simulink model "MOBATSim"  (R2020b)
settings: Solver=FixedStepAuto  StartTime=0.0  StopTime=Sim_t  FixedStep=0.01  MinStep=0.01  RelTol=1e-2
undefined symbols (not defined in the file): meters, noisePower, Sim_Ts, stuckDuration, Vehicle_id, Vehicles
libraries: simulink x32, robotalgslib x11, drivingvehiclecontroller x11, mpcadaslib x1, pid_lib x1
(part 2 of 5)

== system MOBATSim/Vehicle Model 8 ==
  note: Perception
  note: Decision-Making
  note: Control
  Behavioural Planner : MATLABSystem  System=VehicleDrivingMode  Vehicle_id=Vehicle_id  SimulateUsing=Interpreted execution
      mask Type: VehicleDrivingMode
      mask Display:
      | image('MOBATSIM-Icon-Set_7- Behavioural Planner.png');
      | port_label('input',1,'vehicleDetected');
      | port_label('output',1,'SpeedReference');
      | port_label('output',2,'DistanceReference');
      | port_label('output',3,'LeadSpeed');
      | port_label('output',4,'DrivingMode');
      | port_label('output',5,'Dist2Stop');
      | port_label('output',6,'laneChange');
  Longitudinal and Lateral Controllers : Subsystem
  Safety Filter : Subsystem
  Transform to MOBATSim Coordinates : Subsystem
  Vehicle Model - Kinematic 3DOF Single Track : Subsystem  mask{Vehicle_id=Vehicle_id}
      mask prompts: Vehicle_id "Vehicle ID"
      mask Display: image('MOBATSIM-Icon-Set_13- VehicleModel.png'); % Use "Edit Image" on toolstrip to change.
  Vehicle Path Planner : MATLABSystem  System=VehiclePathPlanner_Astar  Vehicle_id=Vehicle_id  SimulateUsing=Interpreted execution
      mask Type: VehiclePathPlanner_Astar
      mask Display:
      | image('MOBATSIM-Icon-Set_8- Navigation.png');
      | port_label('input',1,'CommunicationIDs');
      | port_label('output',1,'waypointReached');
  Vehicle Sensors : MATLABSystem  System=VehicleSensors  Vehicle_id=Vehicle_id  Tsample=Sim_Ts  OffsetTime=0  SimulateUsing=Interpreted execution
      mask Type: VehicleSensors
      mask Display:
      | image('MOBATSIM-Icon-Set_4- Sensor.png');
      | port_label('output',1,'V2VcommIDs');
      | port_label('output',2,'vehicleDetected');
  Vehicle V2I Output : MATLABSystem  System=VehicleV2I_Out  Vehicle_id=Vehicle_id  SimulateUsing=Interpreted execution
      mask Type: VehicleV2I_Out
      mask Display:
      | image('MOBATSIM-Icon-Set_6- V2l.png');
      | port_label('input',1,'waypointReached');
      | port_label('output',1,'V2Idata');
  Position : Outport  VectorParamsAs1DForOutWhenUnconnected=off
  Orientation : Outport  Port=2  VectorParamsAs1DForOutWhenUnconnected=off
  Speed : Outport  Port=3  VectorParamsAs1DForOutWhenUnconnected=off
  V_Network_Out : Outport  Port=4  VectorParamsAs1DForOutWhenUnconnected=off
  wires:
  Vehicle Path Planner/1 -> Vehicle V2I Output/1
  Vehicle Sensors/1 -> Vehicle Path Planner/1
  Vehicle V2I Output/1 -> V_Network_Out/1
  Vehicle Sensors/2 -> Behavioural Planner/1
  Behavioural Planner/1 -> Longitudinal and Lateral Controllers/1(Speed Reference)
  Behavioural Planner/2 -> Longitudinal and Lateral Controllers/2(Inter Vehicular Distance)
  Behavioural Planner/3 -> Longitudinal and Lateral Controllers/3(Lead Speed)
  Behavioural Planner/4 -> Longitudinal and Lateral Controllers/4(drivingMode)
  Behavioural Planner/5 -> Longitudinal and Lateral Controllers/5(Dist2Stop)
  Transform to MOBATSim Coordinates/1(Position) -> Position/1
  Transform to MOBATSim Coordinates/2(Orientation) -> Orientation/1
  Vehicle Model - Kinematic 3DOF Single Track/2(xdot) -> Longitudinal and Lateral Controllers/7(Actual Speed), Speed/1
  Vehicle Model - Kinematic 3DOF Single Track/1(Pose) -> Longitudinal and Lateral Controllers/8(Actual Pose), Transform to MOBATSim Coordinates/1(Pose)
  Longitudinal and Lateral Controllers/1(ref Acc) -> Safety Filter/1(Reference Acceleration)
  Longitudinal and Lateral Controllers/2(ref Steering) -> Safety Filter/2(Reference Steering Angle)
  Safety Filter/1(Steering Angle Cmd) -> Vehicle Model - Kinematic 3DOF Single Track/1(WhlAngF)
  Safety Filter/2(Speed_input) -> Vehicle Model - Kinematic 3DOF Single Track/2(xdotin)
  Behavioural Planner/6 -> Longitudinal and Lateral Controllers/6(laneChange)

== system MOBATSim/Vehicle Model 9 ==
  note: Perception
  note: Decision-Making
  note: Control
  Behavioural Planner : MATLABSystem  System=VehicleDrivingMode  Vehicle_id=Vehicle_id  SimulateUsing=Interpreted execution
      mask Type: VehicleDrivingMode
      mask Display:
      | image('MOBATSIM-Icon-Set_7- Behavioural Planner.png');
      | port_label('input',1,'vehicleDetected');
      | port_label('output',1,'SpeedReference');
      | port_label('output',2,'DistanceReference');
      | port_label('output',3,'LeadSpeed');
      | port_label('output',4,'DrivingMode');
      | port_label('output',5,'Dist2Stop');
      | port_label('output',6,'laneChange');
  Longitudinal and Lateral Controllers : Subsystem
  Safety Filter : Subsystem
  Transform to MOBATSim Coordinates : Subsystem
  Vehicle Model - Kinematic 3DOF Single Track : Subsystem  mask{Vehicle_id=Vehicle_id}
      mask prompts: Vehicle_id "Vehicle ID"
      mask Display: image('MOBATSIM-Icon-Set_13- VehicleModel.png'); % Use "Edit Image" on toolstrip to change.
  Vehicle Path Planner : MATLABSystem  System=VehiclePathPlanner_Astar  Vehicle_id=Vehicle_id  SimulateUsing=Interpreted execution
      mask Type: VehiclePathPlanner_Astar
      mask Display:
      | image('MOBATSIM-Icon-Set_8- Navigation.png');
      | port_label('input',1,'CommunicationIDs');
      | port_label('output',1,'waypointReached');
  Vehicle Sensors : MATLABSystem  System=VehicleSensors  Vehicle_id=Vehicle_id  Tsample=Sim_Ts  OffsetTime=0  SimulateUsing=Interpreted execution
      mask Type: VehicleSensors
      mask Display:
      | image('MOBATSIM-Icon-Set_4- Sensor.png');
      | port_label('output',1,'V2VcommIDs');
      | port_label('output',2,'vehicleDetected');
  Vehicle V2I Output : MATLABSystem  System=VehicleV2I_Out  Vehicle_id=Vehicle_id  SimulateUsing=Interpreted execution
      mask Type: VehicleV2I_Out
      mask Display:
      | image('MOBATSIM-Icon-Set_6- V2l.png');
      | port_label('input',1,'waypointReached');
      | port_label('output',1,'V2Idata');
  Position : Outport  VectorParamsAs1DForOutWhenUnconnected=off
  Orientation : Outport  Port=2  VectorParamsAs1DForOutWhenUnconnected=off
  Speed : Outport  Port=3  VectorParamsAs1DForOutWhenUnconnected=off
  V_Network_Out : Outport  Port=4  VectorParamsAs1DForOutWhenUnconnected=off
  wires:
  Vehicle Path Planner/1 -> Vehicle V2I Output/1
  Vehicle Sensors/1 -> Vehicle Path Planner/1
  Vehicle V2I Output/1 -> V_Network_Out/1
  Vehicle Sensors/2 -> Behavioural Planner/1
  Behavioural Planner/1 -> Longitudinal and Lateral Controllers/1(Speed Reference)
  Behavioural Planner/2 -> Longitudinal and Lateral Controllers/2(Inter Vehicular Distance)
  Behavioural Planner/3 -> Longitudinal and Lateral Controllers/3(Lead Speed)
  Behavioural Planner/4 -> Longitudinal and Lateral Controllers/4(drivingMode)
  Behavioural Planner/5 -> Longitudinal and Lateral Controllers/5(Dist2Stop)
  Transform to MOBATSim Coordinates/1(Position) -> Position/1
  Transform to MOBATSim Coordinates/2(Orientation) -> Orientation/1
  Vehicle Model - Kinematic 3DOF Single Track/2(xdot) -> Longitudinal and Lateral Controllers/7(Actual Speed), Speed/1
  Vehicle Model - Kinematic 3DOF Single Track/1(Pose) -> Longitudinal and Lateral Controllers/8(Actual Pose), Transform to MOBATSim Coordinates/1(Pose)
  Longitudinal and Lateral Controllers/1(ref Acc) -> Safety Filter/1(Reference Acceleration)
  Longitudinal and Lateral Controllers/2(ref Steering) -> Safety Filter/2(Reference Steering Angle)
  Safety Filter/1(Steering Angle Cmd) -> Vehicle Model - Kinematic 3DOF Single Track/1(WhlAngF)
  Safety Filter/2(Speed_input) -> Vehicle Model - Kinematic 3DOF Single Track/2(xdotin)
  Behavioural Planner/6 -> Longitudinal and Lateral Controllers/6(laneChange)

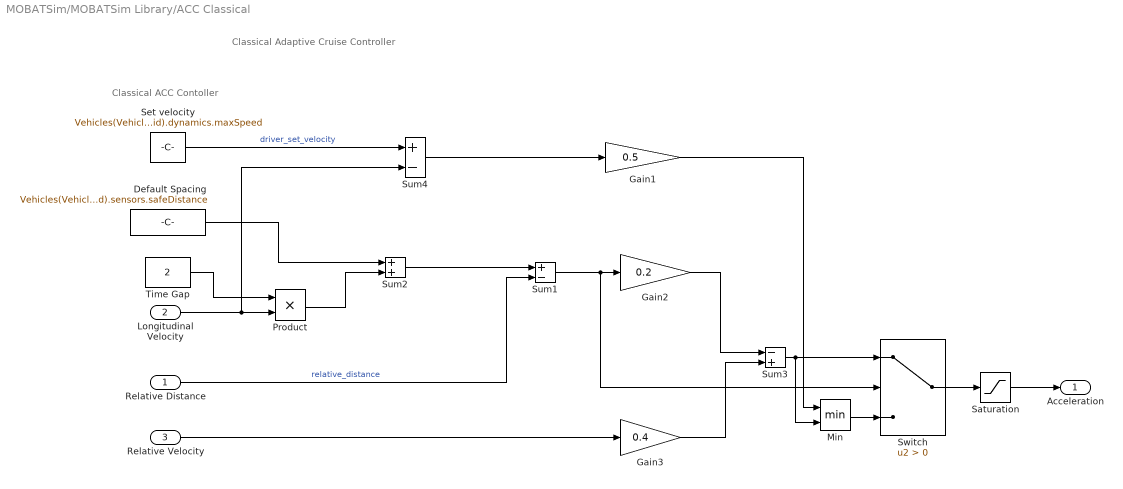
== system MOBATSim/MOBATSim Library/ACC Classical ==
  note: Classical ACC Contoller
  note: Classical Adaptive Cruise Controller
  Relative Distance : Inport
  Longitudinal Velocity : Inport  Port=2
  Relative Velocity : Inport  Port=3
  Default Spacing : Constant  Value=Vehicles(Vehicle_id).sensors.safeDistance  SampleTime=Sim_Ts
  Gain1 : Gain  Gain=0.5
  Gain2 : Gain  Gain=0.2
  Gain3 : Gain  Gain=0.4
  Min : MinMax  Inputs=2
  Product : Product
  Saturation : Saturate  UpperLimit=2  LowerLimit=-3
  Set velocity : Constant  Value=Vehicles(Vehicle_id).dynamics.maxSpeed  SampleTime=Sim_Ts
  Sum1 : Sum  Inputs=+-
  Sum2 : Sum
  Sum3 : Sum  Inputs=-+
  Sum4 : Sum  Inputs=+-
  Switch : Switch  Criteria=u2 > Threshold
  Time Gap : Constant  Value=2  SampleTime=Sim_Ts
  Acceleration : Outport  VectorParamsAs1DForOutWhenUnconnected=off
  wires:
  Longitudinal Velocity/1 -> Product/2, Sum4/2
  Default Spacing/1 -> Sum2/1
  Gain2/1 -> Sum3/1
  Sum4/1 -> Gain1/1
  Min/1 -> Switch/3
  Gain3/1 -> Sum3/2
  Switch/1 -> Saturation/1
  Relative Velocity/1 -> Gain3/1
  Time Gap/1 -> Product/1
  Saturation/1 -> Acceleration/1
  Product/1 -> Sum2/2
  Set velocity/1 -> Sum4/1  "driver_set_velocity"
  Sum3/1 -> Min/2, Switch/1
  Sum1/1 -> Switch/2, Gain2/1
  Gain1/1 -> Min/1
  Relative Distance/1 -> Sum1/2  "relative_distance"
  Sum2/1 -> Sum1/1

== system MOBATSim/MOBATSim Library/Platoon Controller - PID ==
  Inter Vehicular Distance : Inport
  Lead Speed : Inport  Port=2
  Vehicle Speed : Inport  Port=3
  Compare To Constant : simulink/Logic and Bit Operations/Compare To Constant  relop=>  const=2  OutDataTypeStr=uint8
  Constant : Constant  Value=meters
  Gain : Gain  Gain=1.4
  Multiport Switch : MultiPortSwitch  DataPortOrder=Zero-based contiguous  Inputs=2  zeroidx=on
  PID Controller5 : pid_lib/PID Controller  Controller=PID  Form=Parallel  TimeDomain=Continuous-time  UseExternalTs=off  SampleTime=-1  IntegratorMethod=Forward Euler  FilterMethod=Forward Euler  ControllerParametersSource=internal  P=2.0341199375219  I=0.0356576460366845  D=2.08363010404189  UseFilter=on  N=233.214579742572  TunerSelectOption=Transfer Function Based (PID Tuner App)  InitialConditionSource=internal  InitialConditionForIntegrator=0  InitialConditionForFilter=0  DifferentiatorICPrevScaledInput=0  ExternalReset=none  TrackingMode=off  Kt=1  LimitOutput=on  SatLimitsSource=internal  UpperSaturationLimit=100  LowerSaturationLimit=-100  LinearizeAsGain=on  AntiWindupMode=clamping  Kb=1  POutMin=[]  POutMax=[]  IOutMin=[]  IOutMax=[]  DOutMin=[]  DOutMax=[]  NOutMin=[]  NOutMax=[]  SumOutMin=[]  SumOutMax=[]  SaturationOutMin=[]  SaturationOutMax=[]  PParamMin=[]  PParamMax=[]  IParamMin=[]  IParamMax=[]  DParamMin=[]  DParamMax=[]  NParamMin=[]  NParamMax=[]  KbParamMin=[]  KbParamMax=[]  KtParamMin=[]  KtParamMax=[]  KbOutMin=[]  KbOutMax=[]  KtOutMin=[]  KtOutMax=[]  IntegratorOutMin=[]  IntegratorOutMax=[]  FilterOutMin=[]  FilterOutMax=[]  SumI1OutMin=[]  SumI1OutMax=[]  SumI2OutMin=[]  SumI2OutMax=[]  SumI3OutMin=[]  SumI3OutMax=[]  SumI4OutMin=[]  SumI4OutMax=[]  SumDOutMin=[]  SumDOutMax=[]  DifferentiatorOutMin=[]  DifferentiatorOutMax=[]  FilterDiffOutCoefMin=[]  FilterDiffOutCoefMax=[]  ReciprocalOutMin=[]  ReciprocalOutMax=[]  SumDenOutMin=[]  SumDenOutMax=[]  SumNumOutMin=[]  SumNumOutMax=[]  DivideOutMin=[]  DivideOutMax=[]  UdiffTsProdOutMin=[]  UdiffTsProdOutMax=[]  NTsProdOutMin=[]  NTsProdOutMax=[]  UintegralTsProdOutMin=[]  UintegralTsProdOutMax=[]  UngainTsProdOutMin=[]  UngainTsProdOutMax=[]  IntegratorContinuousStateAttributes=''  IntegratorStateMustResolveToSignalObject=off  IntegratorRTWStateStorageClass=Auto  FilterContinuousStateAttributes=''  FilterStateMustResolveToSignalObject=off  FilterRTWStateStorageClass=Auto  ParallelPVariant=InternalParameters  IdealPVariant=Disabled  IVariant=InternalParameters  DVariant=InternalParameters  IntegratorVariant=Continuous  SatVariant=Enabled  AWVariant=ContClampingParallel  PCopyVariant=Disabled  TRVariant=Disabled  FdbkBlocksVariant=Forward  IdealPFdbkVariant=Disabled  SatFdbkVariant=Disabled  DerivativeFilterVariant=ContFilter  NVariant=InternalParameters  NCopyVariant=Disabled  FilterICVariant=InternalICsFilter  IntegratorICVariant=InternalICs  ExternalResetVariant=Disabled  TRSumVariant=Passthrough  SumFdbkVariant=Disabled  SumVariant=Sum_PID  TsampFilterVariant=InternalTs  TsampNgainVariant=Passthrough  TsampIntegralVariant=Passthrough  ExternalSaturationOutDataTypeStr=Inherit: Same as second input
  Sum : Sum  Inputs=|-+
  Sum1 : Sum  Inputs=|++
  Sum2 : Sum  Inputs=|+-
  Transfer Fcn : TransferFcn  Numerator=[0.05]  Denominator=[1 2]
  ref speed : Outport  VectorParamsAs1DForOutWhenUnconnected=off
  wires:
  Transfer Fcn/1 -> PID Controller5/1
  Vehicle Speed/1 -> Gain/1, Sum/1
  PID Controller5/1 -> Multiport Switch/2
  Sum/1 -> Compare To Constant/1
  Multiport Switch/1 -> ref speed/1
  Compare To Constant/1 -> Multiport Switch/1
  Lead Speed/1 -> Sum/2, Multiport Switch/3
  Constant/1 -> Sum1/1
  Sum1/1 -> Sum2/2
  Gain/1 -> Sum1/2
  Sum2/1 -> Transfer Fcn/1
  Inter Vehicular Distance/1 -> Sum2/1

== system MOBATSim/MOBATSim Library/Pure Pursuit with Lane Changing ==
  Speed : Inport
  Pose : Inport  Port=2
  laneChange : Inport  Port=3
  MATLAB System1 : MATLABSystem  System=PurePursuit_WPGenerator  Vehicle_id=Vehicle_id  SimulateUsing=Interpreted execution
      mask Type: PurePursuit_WPGenerator
      mask Display:
      | image('MOBATSIM-Icon-Set_9- PurePursuit WP Generator.png');
      | port_label('input',1,'pose');
      | port_label('input',2,'speed');
      | port_label('input',3,'changeLane');
      | port_label('output',1,'nextWPs');
  Pure Pursuit : robotalgslib/Pure Pursuit  DesiredLinearVelocity=Vehicles(Vehicle_id).dynamics.maxSpeed  MaxAngularVelocity=1  LookaheadDistance=6  TargetDirPort=on  SimulateUsing=Code generation
  Terminator : Terminator
  Terminator1 : Terminator
  Wheel Steering Angle Formulation : Subsystem
  Reference Steering Angle : Outport
  wires:
  laneChange/1 -> MATLAB System1/3
  Speed/1 -> MATLAB System1/2
  Pose/1 -> Pure Pursuit/1, MATLAB System1/1
  Pure Pursuit/1 -> Terminator/1
  Pure Pursuit/2 -> Terminator1/1
  Pure Pursuit/3 -> Wheel Steering Angle Formulation/1(alpha)
  Wheel Steering Angle Formulation/1(referenceYawAngle) -> Reference Steering Angle/1
  MATLAB System1/1 -> Pure Pursuit/2

== system MOBATSim/MOBATSim Library/Stanley Lateral Control ==
  actualSpeed : Inport
  actualPose : Inport  Port=2
  laneChange : Inport  Port=3
  Constant5 : Constant
  Lateral Controller Stanley : drivingvehiclecontroller/Lateral Controller Stanley  ModelType=Kinematic bicycle model  PositionGainF=2.5  PositionGainR=2.5  YawRateGain=0.2  DelayGain=0.2  VehicleMass=1575  Lf=1.2  Lr=1.6  TireStiffness=19000  Wheelbase=3  MaxSteeringAngle=35
      settings: SourceProductBaseCode=DR
  MATLAB System : MATLABSystem  System=Stanley_RefPoseGenerator  Vehicle_id=Vehicle_id  SimulateUsing=Interpreted execution
      mask Type: Stanley_RefPoseGenerator
      mask Display:
      | image('MOBATSIM-Icon-Set_10- Stanley.png');
      | port_label('input',1,'pose');
      | port_label('input',2,'speed');
      | port_label('input',3,'changeLane');
      | port_label('output',1,'poseOut');
      | port_label('output',2,'referencePose');
  SteerCmd_Stanley : Outport
  wires:
  actualPose/1 -> MATLAB System/1
  MATLAB System/1 -> Lateral Controller Stanley/2
  actualSpeed/1 -> Lateral Controller Stanley/3, MATLAB System/2
  Constant5/1 -> Lateral Controller Stanley/4
  MATLAB System/2 -> Lateral Controller Stanley/1
  Lateral Controller Stanley/1 -> SteerCmd_Stanley/1
  laneChange/1 -> MATLAB System/3

== system MOBATSim/Vehicle Model 1/Longitudinal and Lateral Controllers ==
  Speed Reference : Inport
  Inter Vehicular Distance : Inport  Port=2
  Lead Speed : Inport  Port=3
  drivingMode : Inport  Port=4
  Dist2Stop : Inport  Port=5
  laneChange : Inport  Port=6
  Actual Speed : Inport  Port=7
  Actual Pose : Inport  Port=8
  Lateral Motion Control : Subsystem  Variant=on  VariantControlMode=label  LabelModeActiveChoice=STANLEY  mask{modeLateral=STANLEY}
      mask prompts: modeLateral "Lateral Control Mode:"
      mask TypeOptions modeLateral: PURE_PURSUIT | STANLEY
      mask Callback modeLateral: set_param(gcb,'OverrideUsingVariant',get_param(gcb,'modeLateral'));
  Longitudinal Speed Control : Subsystem
  ref Acc : Outport
  ref Steering : Outport  Port=2
  wires:
  laneChange/1 -> Lateral Motion Control/3(changeLane)
  Lateral Motion Control/1(SteerCmd) -> ref Steering/1
  Actual Speed/1 -> Lateral Motion Control/1(speed), Longitudinal Speed Control/6(Actual Speed)
  drivingMode/1 -> Longitudinal Speed Control/4(Driving Mode)
  Longitudinal Speed Control/1(Longitduinal Acceleration Command) -> ref Acc/1
  Dist2Stop/1 -> Longitudinal Speed Control/5(Dist2Stop)
  Inter Vehicular Distance/1 -> Longitudinal Speed Control/2(Inter Vehicular Distance)
  Lead Speed/1 -> Longitudinal Speed Control/3(Lead Speed)
  Speed Reference/1 -> Longitudinal Speed Control/1(Speed Reference)
  Actual Pose/1 -> Lateral Motion Control/2(pose)

== system MOBATSim/Vehicle Model 1/Safety Filter ==
  note: Longitudinal
  Reference Acceleration : Inport
  Reference Steering Angle : Inport  Port=2
  Acceleration to Speed : Integrator  LimitOutput=on  LowerSaturationLimit=0
  MATLAB System : MATLABSystem  System=VehicleSafetyFilter  Vehicle_id=Vehicle_id  SimulateUsing=Interpreted execution
      mask Type: VehicleSafetyFilter
      mask Display:
      | disp('VehicleSafetyFilter');
      | port_label('input',1,'Acc');
      | port_label('input',2,'Steering');
      | port_label('output',1,'Acc');
      | port_label('output',2,'Stop');
      | port_label('output',3,'Steering');
  Product : Product
  Signal Specification : SignalSpecification  Dimensions=1
  Stop Check : simulink/Logic and Bit Operations/Compare To Constant  relop=~=  const=1  OutDataTypeStr=uint8
  Zero-Order Hold : ZeroOrderHold  SampleTime=Sim_Ts
  Steering Angle Cmd : Outport
  Speed_input : Outport  Port=2
  wires:
  Acceleration to Speed/1 -> Signal Specification/1
  Stop Check/1 -> Product/2
  MATLAB System/3 -> Steering Angle Cmd/1
  Signal Specification/1 -> Zero-Order Hold/1
  Reference Acceleration/1 -> MATLAB System/1
  Zero-Order Hold/1 -> Product/1
  Product/1 -> Speed_input/1
  MATLAB System/1 -> Acceleration to Speed/1
  Reference Steering Angle/1 -> MATLAB System/2
  MATLAB System/2 -> Stop Check/1

== system MOBATSim/Vehicle Model 1/Transform to MOBATSim Coordinates ==
  Pose : Inport
  Constant : Constant  Value=0
  Constant1 : Constant
  Constant2 : Constant  Value=0
  Constant3 : Constant  Value=0
  Constant4 : Constant  Value=pi/2
  Gain : Gain  Gain=-1
  Matrix Concatenate : Concatenate  NumInputs=4  ConcatenateDimension=2
  Matrix Concatenate1 : Concatenate  NumInputs=3  ConcatenateDimension=2
  Selector1 : Selector  InputPortWidth=3  IndexOptions=Index vector (dialog)  Indices=[3]  OutputSizes=1
  Selector3 : Selector  InputPortWidth=3  IndexOptions=Index vector (dialog)  Indices=[1]  OutputSizes=1
  Selector4 : Selector  InputPortWidth=3  IndexOptions=Index vector (dialog)  Indices=[2]  OutputSizes=1
  Sum : Sum  Inputs=|++
  Position : Outport
  Orientation : Outport  Port=2
  wires:
  Sum/1 -> Matrix Concatenate/4
  Constant2/1 -> Matrix Concatenate/1
  Constant3/1 -> Matrix Concatenate1/2
  Gain/1 -> Matrix Concatenate1/3
  Constant4/1 -> Sum/2
  Constant1/1 -> Matrix Concatenate/2
  Selector1/1 -> Sum/1
  Constant/1 -> Matrix Concatenate/3
  Matrix Concatenate/1 -> Orientation/1
  Matrix Concatenate1/1 -> Position/1
  Selector4/1 -> Gain/1
  Selector3/1 -> Matrix Concatenate1/1
  Pose/1 -> Selector1/1, Selector4/1, Selector3/1

== system MOBATSim/Vehicle Model 1/Vehicle Model - Kinematic 3DOF Single Track ==
  WhlAngF : Inport
  xdotin : Inport  Port=2
  Delay : Delay  DelayLength=1  SampleTime=Sim_Ts
  Kinematic Bicycle Model : Subsystem
  Selector3 : Selector  InputPortWidth=3  IndexOptions=Index vector (dialog)  Indices=[1]  OutputSizes=1
  Selector4 : Selector  InputPortWidth=3  IndexOptions=Index vector (dialog)  Indices=[2]  OutputSizes=1
  Sqrt : Sqrt  SaturateOnIntegerOverflow=on
  Square : Math  Operator=square  SaturateOnIntegerOverflow=on
  Square1 : Math  Operator=square  SaturateOnIntegerOverflow=on
  Sum1 : Sum  Inputs=|++
  Zero-Order Hold1 : ZeroOrderHold  SampleTime=Sim_Ts
  Zero-Order Hold2 : ZeroOrderHold  SampleTime=Sim_Ts
  Pose : Outport
  xdot : Outport  Port=2
  wires:
  WhlAngF/1 -> Kinematic Bicycle Model/2(Steering Angle)
  xdotin/1 -> Kinematic Bicycle Model/1(v)
  Kinematic Bicycle Model/2(stateDot) -> Zero-Order Hold2/1
  Selector3/1 -> Square/1
  Sum1/1 -> Sqrt/1
  Square1/1 -> Sum1/2
  Selector4/1 -> Square1/1
  Sqrt/1 -> Delay/1
  Square/1 -> Sum1/1
  Delay/1 -> xdot/1
  Kinematic Bicycle Model/1(state) -> Zero-Order Hold1/1
  Zero-Order Hold1/1 -> Pose/1
  Zero-Order Hold2/1 -> Selector3/1, Selector4/1

== system MOBATSim/Vehicle Model 1/noise ==
  In1 : Inport
  Add : Sum
  Band-Limited White Noise : simulink/Sources/Band-Limited White Noise  Cov=[noisePower]  Ts=0.1  seed=[23341]
  Inter Vehicular Distance : Outport
  wires:
  In1/1 -> Add/1
  Band-Limited White Noise/1 -> Add/2
  Add/1 -> Inter Vehicular Distance/1

== system MOBATSim/Vehicle Model 1/stuck_at ==
  In1 : Inport
  Data Store Memory : DataStoreMemory  ReadBeforeWriteMsg=warning  WriteAfterWriteMsg=warning  WriteAfterReadMsg=warning  ShowAdditionalParam=off  OutDataTypeStr=double
  Digital Clock1 : DigitalClock  SampleTime=Sim_Ts
  MATLAB Function : MATLAB Function  TreatAsAtomicUnit=on
  Scope : Scope  NumInputPorts=2
  stuckDuration : Constant  Value=stuckDuration
  stuck_start : Constant  Value=26
  Speed Reference : Outport
  wires:
  In1/1 -> MATLAB Function/1(u)
  MATLAB Function/1(y) -> Speed Reference/1
  Digital Clock1/1 -> MATLAB Function/4(t)
  stuck_start/1 -> MATLAB Function/2(stuck_start)
  stuckDuration/1 -> MATLAB Function/3(stuck_duration)
  MATLAB Function/2(stuck_value1) -> Scope/1
  MATLAB Function/3(trigger) -> Scope/2

== system MOBATSim/Vehicle Model 10/Longitudinal and Lateral Controllers ==
  Speed Reference : Inport
  Inter Vehicular Distance : Inport  Port=2
  Lead Speed : Inport  Port=3
  drivingMode : Inport  Port=4
  Dist2Stop : Inport  Port=5
  laneChange : Inport  Port=6
  Actual Speed : Inport  Port=7
  Actual Pose : Inport  Port=8
  Lateral Motion Control : Subsystem  Variant=on  VariantControlMode=label  LabelModeActiveChoice=STANLEY  mask{modeLateral=STANLEY}
      mask prompts: modeLateral "Lateral Control Mode:"
      mask TypeOptions modeLateral: PURE_PURSUIT | STANLEY
      mask Callback modeLateral: set_param(gcb,'OverrideUsingVariant',get_param(gcb,'modeLateral'));
  Longitudinal Speed Control : Subsystem
  ref Acc : Outport
  ref Steering : Outport  Port=2
  wires:
  laneChange/1 -> Lateral Motion Control/3(changeLane)
  Lateral Motion Control/1(SteerCmd) -> ref Steering/1
  Actual Speed/1 -> Lateral Motion Control/1(speed), Longitudinal Speed Control/6(Actual Speed)
  drivingMode/1 -> Longitudinal Speed Control/4(Driving Mode)
  Longitudinal Speed Control/1(Longitduinal Acceleration Command) -> ref Acc/1
  Dist2Stop/1 -> Longitudinal Speed Control/5(Dist2Stop)
  Inter Vehicular Distance/1 -> Longitudinal Speed Control/2(Inter Vehicular Distance)
  Lead Speed/1 -> Longitudinal Speed Control/3(Lead Speed)
  Speed Reference/1 -> Longitudinal Speed Control/1(Speed Reference)
  Actual Pose/1 -> Lateral Motion Control/2(pose)

== system MOBATSim/Vehicle Model 10/Safety Filter ==
  note: Longitudinal
  Reference Acceleration : Inport
  Reference Steering Angle : Inport  Port=2
  Acceleration to Speed : Integrator  LimitOutput=on  LowerSaturationLimit=0
  MATLAB System : MATLABSystem  System=VehicleSafetyFilter  Vehicle_id=Vehicle_id  SimulateUsing=Interpreted execution
      mask Type: VehicleSafetyFilter
      mask Display:
      | disp('VehicleSafetyFilter');
      | port_label('input',1,'Acc');
      | port_label('input',2,'Steering');
      | port_label('output',1,'Acc');
      | port_label('output',2,'Stop');
      | port_label('output',3,'Steering');
  Product : Product
  Signal Specification : SignalSpecification  Dimensions=1
  Stop Check : simulink/Logic and Bit Operations/Compare To Constant  relop=~=  const=1  OutDataTypeStr=uint8
  Zero-Order Hold : ZeroOrderHold  SampleTime=Sim_Ts
  Steering Angle Cmd : Outport
  Speed_input : Outport  Port=2
  wires:
  Acceleration to Speed/1 -> Signal Specification/1
  Stop Check/1 -> Product/2
  MATLAB System/3 -> Steering Angle Cmd/1
  Signal Specification/1 -> Zero-Order Hold/1
  Reference Acceleration/1 -> MATLAB System/1
  Zero-Order Hold/1 -> Product/1
  Product/1 -> Speed_input/1
  MATLAB System/1 -> Acceleration to Speed/1
  Reference Steering Angle/1 -> MATLAB System/2
  MATLAB System/2 -> Stop Check/1

== system MOBATSim/Vehicle Model 10/Transform to MOBATSim Coordinates ==
  Pose : Inport
  Constant : Constant  Value=0
  Constant1 : Constant
  Constant2 : Constant  Value=0
  Constant3 : Constant  Value=0
  Constant4 : Constant  Value=pi/2
  Gain : Gain  Gain=-1
  Matrix Concatenate : Concatenate  NumInputs=4  ConcatenateDimension=2
  Matrix Concatenate1 : Concatenate  NumInputs=3  ConcatenateDimension=2
  Selector1 : Selector  InputPortWidth=3  IndexOptions=Index vector (dialog)  Indices=[3]  OutputSizes=1
  Selector3 : Selector  InputPortWidth=3  IndexOptions=Index vector (dialog)  Indices=[1]  OutputSizes=1
  Selector4 : Selector  InputPortWidth=3  IndexOptions=Index vector (dialog)  Indices=[2]  OutputSizes=1
  Sum : Sum  Inputs=|++
  Position : Outport
  Orientation : Outport  Port=2
  wires:
  Sum/1 -> Matrix Concatenate/4
  Constant2/1 -> Matrix Concatenate/1
  Constant3/1 -> Matrix Concatenate1/2
  Gain/1 -> Matrix Concatenate1/3
  Constant4/1 -> Sum/2
  Constant1/1 -> Matrix Concatenate/2
  Selector1/1 -> Sum/1
  Constant/1 -> Matrix Concatenate/3
  Matrix Concatenate/1 -> Orientation/1
  Matrix Concatenate1/1 -> Position/1
  Selector4/1 -> Gain/1
  Selector3/1 -> Matrix Concatenate1/1
  Pose/1 -> Selector1/1, Selector4/1, Selector3/1

== system MOBATSim/Vehicle Model 10/Vehicle Model - Kinematic 3DOF Single Track ==
  WhlAngF : Inport
  xdotin : Inport  Port=2
  Delay : Delay  DelayLength=1  SampleTime=Sim_Ts
  Kinematic Bicycle Model : Subsystem
  Selector3 : Selector  InputPortWidth=3  IndexOptions=Index vector (dialog)  Indices=[1]  OutputSizes=1
  Selector4 : Selector  InputPortWidth=3  IndexOptions=Index vector (dialog)  Indices=[2]  OutputSizes=1
  Sqrt : Sqrt  SaturateOnIntegerOverflow=on
  Square : Math  Operator=square  SaturateOnIntegerOverflow=on
  Square1 : Math  Operator=square  SaturateOnIntegerOverflow=on
  Sum1 : Sum  Inputs=|++
  Zero-Order Hold1 : ZeroOrderHold  SampleTime=Sim_Ts
  Zero-Order Hold2 : ZeroOrderHold  SampleTime=Sim_Ts
  Pose : Outport
  xdot : Outport  Port=2
  wires:
  WhlAngF/1 -> Kinematic Bicycle Model/2(Steering Angle)
  xdotin/1 -> Kinematic Bicycle Model/1(v)
  Kinematic Bicycle Model/2(stateDot) -> Zero-Order Hold2/1
  Selector3/1 -> Square/1
  Sum1/1 -> Sqrt/1
  Square1/1 -> Sum1/2
  Selector4/1 -> Square1/1
  Sqrt/1 -> Delay/1
  Square/1 -> Sum1/1
  Delay/1 -> xdot/1
  Kinematic Bicycle Model/1(state) -> Zero-Order Hold1/1
  Zero-Order Hold1/1 -> Pose/1
  Zero-Order Hold2/1 -> Selector3/1, Selector4/1

== system MOBATSim/Vehicle Model 2/Longitudinal and Lateral Controllers ==
  Speed Reference : Inport
  Inter Vehicular Distance : Inport  Port=2
  Lead Speed : Inport  Port=3
  Driving Mode : Inport  Port=4
  Dist2Stop : Inport  Port=5
  laneChange : Inport  Port=6
  Actual Pose : Inport  Port=7
  Actual Speed : Inport  Port=8
  Lateral Motion Control : Subsystem  Variant=on  VariantControlMode=label  LabelModeActiveChoice=STANLEY  mask{modeLateral=STANLEY}
      mask prompts: modeLateral "Lateral Control Mode:"
      mask TypeOptions modeLateral: PURE_PURSUIT | STANLEY
      mask Callback modeLateral: set_param(gcb,'OverrideUsingVariant',get_param(gcb,'modeLateral'));
  Longitudinal Speed Control : Subsystem
  Longitudinal Acceleration Cmd : Outport
  Reference Steering Angle : Outport  Port=2
  wires:
  Driving Mode/1 -> Longitudinal Speed Control/4(Driving Mode)
  Inter Vehicular Distance/1 -> Longitudinal Speed Control/2(Inter Vehicular Distance)
  Speed Reference/1 -> Longitudinal Speed Control/1(Speed Reference)
  Lead Speed/1 -> Longitudinal Speed Control/3(Lead Speed)
  Dist2Stop/1 -> Longitudinal Speed Control/5(Dist2Stop)
  Actual Speed/1 -> Lateral Motion Control/1(speed), Longitudinal Speed Control/6(Actual Speed)
  Longitudinal Speed Control/1(Longitduinal Acceleration Command) -> Longitudinal Acceleration Cmd/1
  laneChange/1 -> Lateral Motion Control/3(changeLane)
  Actual Pose/1 -> Lateral Motion Control/2(pose)
  Lateral Motion Control/1(SteerCmd) -> Reference Steering Angle/1

== system MOBATSim/Vehicle Model 2/Safety Filter ==
  note: Longitudinal
  Reference Acceleration : Inport
  Reference Steering Angle : Inport  Port=2
  Acceleration to Speed : Integrator  LimitOutput=on  UpperSaturationLimit=Vehicles(Vehicle_id).dynamics.maxSpeed  LowerSaturationLimit=0
  MATLAB System : MATLABSystem  System=VehicleSafetyFilter  Vehicle_id=Vehicle_id  SimulateUsing=Interpreted execution
      mask Type: VehicleSafetyFilter
      mask Display:
      | disp('VehicleSafetyFilter');
      | port_label('input',1,'Acc');
      | port_label('input',2,'Steering');
      | port_label('output',1,'Acc');
      | port_label('output',2,'Stop');
      | port_label('output',3,'Steering');
  Product : Product
  Signal Specification : SignalSpecification  Dimensions=1
  Stop Check : simulink/Logic and Bit Operations/Compare To Constant  relop=~=  const=1  OutDataTypeStr=uint8
  Zero-Order Hold : ZeroOrderHold  SampleTime=Sim_Ts
  Speed_input : Outport
  Steering Angle Cmd : Outport  Port=2
  wires:
  Acceleration to Speed/1 -> Signal Specification/1
  Stop Check/1 -> Product/2
  Signal Specification/1 -> Zero-Order Hold/1
  Reference Acceleration/1 -> MATLAB System/1
  Zero-Order Hold/1 -> Product/1
  Product/1 -> Speed_input/1
  MATLAB System/1 -> Acceleration to Speed/1
  Reference Steering Angle/1 -> MATLAB System/2
  MATLAB System/3 -> Steering Angle Cmd/1
  MATLAB System/2 -> Stop Check/1

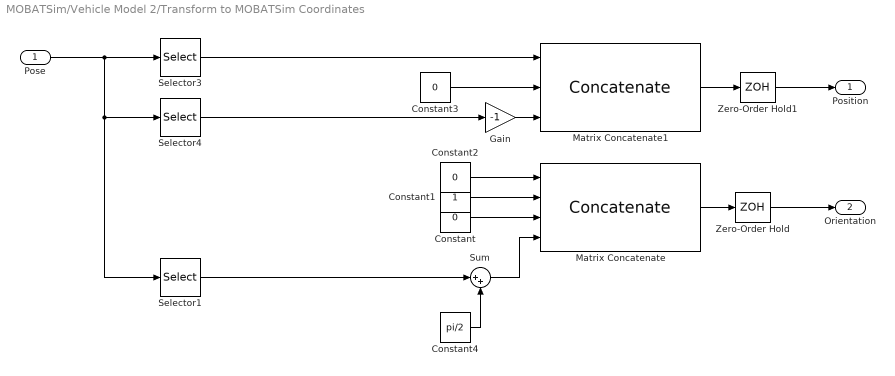
== system MOBATSim/Vehicle Model 2/Transform to MOBATSim Coordinates ==
  Pose : Inport
  Constant : Constant  Value=0
  Constant1 : Constant
  Constant2 : Constant  Value=0
  Constant3 : Constant  Value=0
  Constant4 : Constant  Value=pi/2
  Gain : Gain  Gain=-1
  Matrix Concatenate : Concatenate  NumInputs=4  ConcatenateDimension=2
  Matrix Concatenate1 : Concatenate  NumInputs=3  ConcatenateDimension=2
  Selector1 : Selector  InputPortWidth=3  IndexOptions=Index vector (dialog)  Indices=[3]  OutputSizes=1
  Selector3 : Selector  InputPortWidth=3  IndexOptions=Index vector (dialog)  Indices=[1]  OutputSizes=1
  Selector4 : Selector  InputPortWidth=3  IndexOptions=Index vector (dialog)  Indices=[2]  OutputSizes=1
  Sum : Sum  Inputs=|++
  Zero-Order Hold : ZeroOrderHold  SampleTime=Sim_Ts
  Zero-Order Hold1 : ZeroOrderHold  SampleTime=Sim_Ts
  Position : Outport
  Orientation : Outport  Port=2
  wires:
  Sum/1 -> Matrix Concatenate/4
  Constant2/1 -> Matrix Concatenate/1
  Matrix Concatenate/1 -> Zero-Order Hold/1
  Constant3/1 -> Matrix Concatenate1/2
  Gain/1 -> Matrix Concatenate1/3
  Constant4/1 -> Sum/2
  Constant1/1 -> Matrix Concatenate/2
  Matrix Concatenate1/1 -> Zero-Order Hold1/1
  Selector1/1 -> Sum/1
  Constant/1 -> Matrix Concatenate/3
  Zero-Order Hold/1 -> Orientation/1
  Zero-Order Hold1/1 -> Position/1
  Selector4/1 -> Gain/1
  Selector3/1 -> Matrix Concatenate1/1
  Pose/1 -> Selector1/1, Selector4/1, Selector3/1

== system MOBATSim/Vehicle Model 2/Vehicle Model - Kinematic 3DOF Single Track ==
  Longitudinal Speed : Inport
  Steering Angle : Inport  Port=2
  Delay : Delay  DelayLength=1  SampleTime=Sim_Ts
  Kinematic Bicycle Model : Subsystem
  Selector3 : Selector  InputPortWidth=3  IndexOptions=Index vector (dialog)  Indices=[1]  OutputSizes=1
  Selector4 : Selector  InputPortWidth=3  IndexOptions=Index vector (dialog)  Indices=[2]  OutputSizes=1
  Sqrt : Sqrt  SaturateOnIntegerOverflow=on
  Square : Math  Operator=square  SaturateOnIntegerOverflow=on
  Square1 : Math  Operator=square  SaturateOnIntegerOverflow=on
  Sum1 : Sum  Inputs=|++
  Zero-Order Hold1 : ZeroOrderHold  SampleTime=Sim_Ts
  Zero-Order Hold2 : ZeroOrderHold  SampleTime=Sim_Ts
  Pose : Outport
  Speed : Outport  Port=2
  wires:
  Delay/1 -> Speed/1
  Kinematic Bicycle Model/1(state) -> Zero-Order Hold1/1
  Selector4/1 -> Square1/1
  Longitudinal Speed/1 -> Kinematic Bicycle Model/1(v)
  Steering Angle/1 -> Kinematic Bicycle Model/2(Steering Angle)
  Sum1/1 -> Sqrt/1
  Sqrt/1 -> Delay/1
  Square/1 -> Sum1/1
  Square1/1 -> Sum1/2
  Selector3/1 -> Square/1
  Kinematic Bicycle Model/2(stateDot) -> Zero-Order Hold2/1
  Zero-Order Hold1/1 -> Pose/1
  Zero-Order Hold2/1 -> Selector4/1, Selector3/1

== system MOBATSim/Vehicle Model 3/Longitudinal and Lateral Controllers ==
  Speed Reference : Inport
  Inter Vehicular Distance : Inport  Port=2
  Lead Speed : Inport  Port=3
  drivingMode : Inport  Port=4
  Dist2Stop : Inport  Port=5
  laneChange : Inport  Port=6
  Actual Speed : Inport  Port=7
  Actual Pose : Inport  Port=8
  Lateral Motion Control : Subsystem  Variant=on  VariantControlMode=label  LabelModeActiveChoice=STANLEY  mask{modeLateral=STANLEY}
      mask prompts: modeLateral "Lateral Control Mode:"
      mask TypeOptions modeLateral: PURE_PURSUIT | STANLEY
      mask Callback modeLateral: set_param(gcb,'OverrideUsingVariant',get_param(gcb,'modeLateral'));
  Longitudinal Speed Control : Subsystem
  ref Acc : Outport
  ref Steering : Outport  Port=2
  wires:
  laneChange/1 -> Lateral Motion Control/3(changeLane)
  Lateral Motion Control/1(SteerCmd) -> ref Steering/1
  Actual Speed/1 -> Lateral Motion Control/1(speed), Longitudinal Speed Control/6(Actual Speed)
  drivingMode/1 -> Longitudinal Speed Control/4(Driving Mode)
  Longitudinal Speed Control/1(Longitduinal Acceleration Command) -> ref Acc/1
  Dist2Stop/1 -> Longitudinal Speed Control/5(Dist2Stop)
  Inter Vehicular Distance/1 -> Longitudinal Speed Control/2(Inter Vehicular Distance)
  Lead Speed/1 -> Longitudinal Speed Control/3(Lead Speed)
  Speed Reference/1 -> Longitudinal Speed Control/1(Speed Reference)
  Actual Pose/1 -> Lateral Motion Control/2(pose)

== system MOBATSim/Vehicle Model 3/Safety Filter ==
  note: Longitudinal
  Reference Acceleration : Inport
  Reference Steering Angle : Inport  Port=2
  Acceleration to Speed : Integrator  LimitOutput=on  LowerSaturationLimit=0
  MATLAB System : MATLABSystem  System=VehicleSafetyFilter  Vehicle_id=Vehicle_id  SimulateUsing=Interpreted execution
      mask Type: VehicleSafetyFilter
      mask Display:
      | disp('VehicleSafetyFilter');
      | port_label('input',1,'Acc');
      | port_label('input',2,'Steering');
      | port_label('output',1,'Acc');
      | port_label('output',2,'Stop');
      | port_label('output',3,'Steering');
  Product : Product
  Signal Specification : SignalSpecification  Dimensions=1
  Stop Check : simulink/Logic and Bit Operations/Compare To Constant  relop=~=  const=1  OutDataTypeStr=uint8
  Zero-Order Hold : ZeroOrderHold  SampleTime=Sim_Ts
  Steering Angle Cmd : Outport
  Speed_input : Outport  Port=2
  wires:
  Acceleration to Speed/1 -> Signal Specification/1
  Stop Check/1 -> Product/2
  MATLAB System/3 -> Steering Angle Cmd/1
  Signal Specification/1 -> Zero-Order Hold/1
  Reference Acceleration/1 -> MATLAB System/1
  Zero-Order Hold/1 -> Product/1
  Product/1 -> Speed_input/1
  MATLAB System/1 -> Acceleration to Speed/1
  Reference Steering Angle/1 -> MATLAB System/2
  MATLAB System/2 -> Stop Check/1

== system MOBATSim/Vehicle Model 3/Transform to MOBATSim Coordinates ==
  Pose : Inport
  Constant : Constant  Value=0
  Constant1 : Constant
  Constant2 : Constant  Value=0
  Constant3 : Constant  Value=0
  Constant4 : Constant  Value=pi/2
  Gain : Gain  Gain=-1
  Matrix Concatenate : Concatenate  NumInputs=4  ConcatenateDimension=2
  Matrix Concatenate1 : Concatenate  NumInputs=3  ConcatenateDimension=2
  Selector1 : Selector  InputPortWidth=3  IndexOptions=Index vector (dialog)  Indices=[3]  OutputSizes=1
  Selector3 : Selector  InputPortWidth=3  IndexOptions=Index vector (dialog)  Indices=[1]  OutputSizes=1
  Selector4 : Selector  InputPortWidth=3  IndexOptions=Index vector (dialog)  Indices=[2]  OutputSizes=1
  Sum : Sum  Inputs=|++
  Position : Outport
  Orientation : Outport  Port=2
  wires:
  Sum/1 -> Matrix Concatenate/4
  Constant2/1 -> Matrix Concatenate/1
  Constant3/1 -> Matrix Concatenate1/2
  Gain/1 -> Matrix Concatenate1/3
  Constant4/1 -> Sum/2
  Constant1/1 -> Matrix Concatenate/2
  Selector1/1 -> Sum/1
  Constant/1 -> Matrix Concatenate/3
  Matrix Concatenate/1 -> Orientation/1
  Matrix Concatenate1/1 -> Position/1
  Selector4/1 -> Gain/1
  Selector3/1 -> Matrix Concatenate1/1
  Pose/1 -> Selector1/1, Selector4/1, Selector3/1

== system MOBATSim/Vehicle Model 3/Vehicle Model - Kinematic 3DOF Single Track ==
  WhlAngF : Inport
  xdotin : Inport  Port=2
  Delay : Delay  DelayLength=1  SampleTime=Sim_Ts
  Kinematic Bicycle Model : Subsystem
  Selector3 : Selector  InputPortWidth=3  IndexOptions=Index vector (dialog)  Indices=[1]  OutputSizes=1
  Selector4 : Selector  InputPortWidth=3  IndexOptions=Index vector (dialog)  Indices=[2]  OutputSizes=1
  Sqrt : Sqrt  SaturateOnIntegerOverflow=on
  Square : Math  Operator=square  SaturateOnIntegerOverflow=on
  Square1 : Math  Operator=square  SaturateOnIntegerOverflow=on
  Sum1 : Sum  Inputs=|++
  Zero-Order Hold1 : ZeroOrderHold  SampleTime=Sim_Ts
  Zero-Order Hold2 : ZeroOrderHold  SampleTime=Sim_Ts
  Pose : Outport
  xdot : Outport  Port=2
  wires:
  WhlAngF/1 -> Kinematic Bicycle Model/2(Steering Angle)
  xdotin/1 -> Kinematic Bicycle Model/1(v)
  Kinematic Bicycle Model/2(stateDot) -> Zero-Order Hold2/1
  Selector3/1 -> Square/1
  Sum1/1 -> Sqrt/1
  Square1/1 -> Sum1/2
  Selector4/1 -> Square1/1
  Sqrt/1 -> Delay/1
  Square/1 -> Sum1/1
  Delay/1 -> xdot/1
  Kinematic Bicycle Model/1(state) -> Zero-Order Hold1/1
  Zero-Order Hold1/1 -> Pose/1
  Zero-Order Hold2/1 -> Selector3/1, Selector4/1

== system MOBATSim/Vehicle Model 4/Longitudinal and Lateral Controllers ==
  Speed Reference : Inport
  Inter Vehicular Distance : Inport  Port=2
  Lead Speed : Inport  Port=3
  drivingMode : Inport  Port=4
  Dist2Stop : Inport  Port=5
  laneChange : Inport  Port=6
  Actual Speed : Inport  Port=7
  Actual Pose : Inport  Port=8
  Lateral Motion Control : Subsystem  Variant=on  VariantControlMode=label  LabelModeActiveChoice=STANLEY  mask{modeLateral=STANLEY}
      mask prompts: modeLateral "Lateral Control Mode:"
      mask TypeOptions modeLateral: PURE_PURSUIT | STANLEY
      mask Callback modeLateral: set_param(gcb,'OverrideUsingVariant',get_param(gcb,'modeLateral'));
  Longitudinal Speed Control : Subsystem
  ref Acc : Outport
  ref Steering : Outport  Port=2
  wires:
  laneChange/1 -> Lateral Motion Control/3(changeLane)
  Lateral Motion Control/1(SteerCmd) -> ref Steering/1
  Actual Speed/1 -> Lateral Motion Control/1(speed), Longitudinal Speed Control/6(Actual Speed)
  drivingMode/1 -> Longitudinal Speed Control/4(Driving Mode)
  Longitudinal Speed Control/1(Longitduinal Acceleration Command) -> ref Acc/1
  Dist2Stop/1 -> Longitudinal Speed Control/5(Dist2Stop)
  Inter Vehicular Distance/1 -> Longitudinal Speed Control/2(Inter Vehicular Distance)
  Lead Speed/1 -> Longitudinal Speed Control/3(Lead Speed)
  Speed Reference/1 -> Longitudinal Speed Control/1(Speed Reference)
  Actual Pose/1 -> Lateral Motion Control/2(pose)

== system MOBATSim/Vehicle Model 4/Safety Filter ==
  note: Longitudinal
  Reference Acceleration : Inport
  Reference Steering Angle : Inport  Port=2
  Acceleration to Speed : Integrator  LimitOutput=on  LowerSaturationLimit=0
  MATLAB System : MATLABSystem  System=VehicleSafetyFilter  Vehicle_id=Vehicle_id  SimulateUsing=Interpreted execution
      mask Type: VehicleSafetyFilter
      mask Display:
      | disp('VehicleSafetyFilter');
      | port_label('input',1,'Acc');
      | port_label('input',2,'Steering');
      | port_label('output',1,'Acc');
      | port_label('output',2,'Stop');
      | port_label('output',3,'Steering');
  Product : Product
  Signal Specification : SignalSpecification  Dimensions=1
  Stop Check : simulink/Logic and Bit Operations/Compare To Constant  relop=~=  const=1  OutDataTypeStr=uint8
  Zero-Order Hold : ZeroOrderHold  SampleTime=Sim_Ts
  Steering Angle Cmd : Outport
  Speed_input : Outport  Port=2
  wires:
  Acceleration to Speed/1 -> Signal Specification/1
  Stop Check/1 -> Product/2
  MATLAB System/3 -> Steering Angle Cmd/1
  Signal Specification/1 -> Zero-Order Hold/1
  Reference Acceleration/1 -> MATLAB System/1
  Zero-Order Hold/1 -> Product/1
  Product/1 -> Speed_input/1
  MATLAB System/1 -> Acceleration to Speed/1
  Reference Steering Angle/1 -> MATLAB System/2
  MATLAB System/2 -> Stop Check/1

== system MOBATSim/Vehicle Model 4/Transform to MOBATSim Coordinates ==
  Pose : Inport
  Constant : Constant  Value=0
  Constant1 : Constant
  Constant2 : Constant  Value=0
  Constant3 : Constant  Value=0
  Constant4 : Constant  Value=pi/2
  Gain : Gain  Gain=-1
  Matrix Concatenate : Concatenate  NumInputs=4  ConcatenateDimension=2
  Matrix Concatenate1 : Concatenate  NumInputs=3  ConcatenateDimension=2
  Selector1 : Selector  InputPortWidth=3  IndexOptions=Index vector (dialog)  Indices=[3]  OutputSizes=1
  Selector3 : Selector  InputPortWidth=3  IndexOptions=Index vector (dialog)  Indices=[1]  OutputSizes=1
  Selector4 : Selector  InputPortWidth=3  IndexOptions=Index vector (dialog)  Indices=[2]  OutputSizes=1
  Sum : Sum  Inputs=|++
  Position : Outport
  Orientation : Outport  Port=2
  wires:
  Sum/1 -> Matrix Concatenate/4
  Constant2/1 -> Matrix Concatenate/1
  Constant3/1 -> Matrix Concatenate1/2
  Gain/1 -> Matrix Concatenate1/3
  Constant4/1 -> Sum/2
  Constant1/1 -> Matrix Concatenate/2
  Selector1/1 -> Sum/1
  Constant/1 -> Matrix Concatenate/3
  Matrix Concatenate/1 -> Orientation/1
  Matrix Concatenate1/1 -> Position/1
  Selector4/1 -> Gain/1
  Selector3/1 -> Matrix Concatenate1/1
  Pose/1 -> Selector1/1, Selector4/1, Selector3/1

== system MOBATSim/Vehicle Model 4/Vehicle Model - Kinematic 3DOF Single Track ==
  WhlAngF : Inport
  xdotin : Inport  Port=2
  Delay : Delay  DelayLength=1  SampleTime=Sim_Ts
  Kinematic Bicycle Model : Subsystem
  Selector3 : Selector  InputPortWidth=3  IndexOptions=Index vector (dialog)  Indices=[1]  OutputSizes=1
  Selector4 : Selector  InputPortWidth=3  IndexOptions=Index vector (dialog)  Indices=[2]  OutputSizes=1
  Sqrt : Sqrt  SaturateOnIntegerOverflow=on
  Square : Math  Operator=square  SaturateOnIntegerOverflow=on
  Square1 : Math  Operator=square  SaturateOnIntegerOverflow=on
  Sum1 : Sum  Inputs=|++
  Zero-Order Hold1 : ZeroOrderHold  SampleTime=Sim_Ts
  Zero-Order Hold2 : ZeroOrderHold  SampleTime=Sim_Ts
  Pose : Outport
  xdot : Outport  Port=2
  wires:
  WhlAngF/1 -> Kinematic Bicycle Model/2(Steering Angle)
  xdotin/1 -> Kinematic Bicycle Model/1(v)
  Kinematic Bicycle Model/2(stateDot) -> Zero-Order Hold2/1
  Selector3/1 -> Square/1
  Sum1/1 -> Sqrt/1
  Square1/1 -> Sum1/2
  Selector4/1 -> Square1/1
  Sqrt/1 -> Delay/1
  Square/1 -> Sum1/1
  Delay/1 -> xdot/1
  Kinematic Bicycle Model/1(state) -> Zero-Order Hold1/1
  Zero-Order Hold1/1 -> Pose/1
  Zero-Order Hold2/1 -> Selector3/1, Selector4/1

== system MOBATSim/Vehicle Model 5/Longitudinal and Lateral Controllers ==
  Speed Reference : Inport
  Inter Vehicular Distance : Inport  Port=2
  Lead Speed : Inport  Port=3
  drivingMode : Inport  Port=4
  Dist2Stop : Inport  Port=5
  laneChange : Inport  Port=6
  Actual Speed : Inport  Port=7
  Actual Pose : Inport  Port=8
  Lateral Motion Control : Subsystem  Variant=on  VariantControlMode=label  LabelModeActiveChoice=STANLEY  mask{modeLateral=STANLEY}
      mask prompts: modeLateral "Lateral Control Mode:"
      mask TypeOptions modeLateral: PURE_PURSUIT | STANLEY
      mask Callback modeLateral: set_param(gcb,'OverrideUsingVariant',get_param(gcb,'modeLateral'));
  Longitudinal Speed Control : Subsystem
  ref Acc : Outport
  ref Steering : Outport  Port=2
  wires:
  laneChange/1 -> Lateral Motion Control/3(changeLane)
  Lateral Motion Control/1(SteerCmd) -> ref Steering/1
  Actual Speed/1 -> Lateral Motion Control/1(speed), Longitudinal Speed Control/6(Actual Speed)
  drivingMode/1 -> Longitudinal Speed Control/4(Driving Mode)
  Longitudinal Speed Control/1(Longitduinal Acceleration Command) -> ref Acc/1
  Dist2Stop/1 -> Longitudinal Speed Control/5(Dist2Stop)
  Inter Vehicular Distance/1 -> Longitudinal Speed Control/2(Inter Vehicular Distance)
  Lead Speed/1 -> Longitudinal Speed Control/3(Lead Speed)
  Speed Reference/1 -> Longitudinal Speed Control/1(Speed Reference)
  Actual Pose/1 -> Lateral Motion Control/2(pose)

== system MOBATSim/Vehicle Model 5/Safety Filter ==
  note: Longitudinal
  Reference Acceleration : Inport
  Reference Steering Angle : Inport  Port=2
  Acceleration to Speed : Integrator  LimitOutput=on  LowerSaturationLimit=0
  MATLAB System : MATLABSystem  System=VehicleSafetyFilter  Vehicle_id=Vehicle_id  SimulateUsing=Interpreted execution
      mask Type: VehicleSafetyFilter
      mask Display:
      | disp('VehicleSafetyFilter');
      | port_label('input',1,'Acc');
      | port_label('input',2,'Steering');
      | port_label('output',1,'Acc');
      | port_label('output',2,'Stop');
      | port_label('output',3,'Steering');
  Product : Product
  Signal Specification : SignalSpecification  Dimensions=1
  Stop Check : simulink/Logic and Bit Operations/Compare To Constant  relop=~=  const=1  OutDataTypeStr=uint8
  Zero-Order Hold : ZeroOrderHold  SampleTime=Sim_Ts
  Steering Angle Cmd : Outport
  Speed_input : Outport  Port=2
  wires:
  Acceleration to Speed/1 -> Signal Specification/1
  Stop Check/1 -> Product/2
  MATLAB System/3 -> Steering Angle Cmd/1
  Signal Specification/1 -> Zero-Order Hold/1
  Reference Acceleration/1 -> MATLAB System/1
  Zero-Order Hold/1 -> Product/1
  Product/1 -> Speed_input/1
  MATLAB System/1 -> Acceleration to Speed/1
  Reference Steering Angle/1 -> MATLAB System/2
  MATLAB System/2 -> Stop Check/1

== system MOBATSim/Vehicle Model 5/Transform to MOBATSim Coordinates ==
  Pose : Inport
  Constant : Constant  Value=0
  Constant1 : Constant
  Constant2 : Constant  Value=0
  Constant3 : Constant  Value=0
  Constant4 : Constant  Value=pi/2
  Gain : Gain  Gain=-1
  Matrix Concatenate : Concatenate  NumInputs=4  ConcatenateDimension=2
  Matrix Concatenate1 : Concatenate  NumInputs=3  ConcatenateDimension=2
  Selector1 : Selector  InputPortWidth=3  IndexOptions=Index vector (dialog)  Indices=[3]  OutputSizes=1
  Selector3 : Selector  InputPortWidth=3  IndexOptions=Index vector (dialog)  Indices=[1]  OutputSizes=1
  Selector4 : Selector  InputPortWidth=3  IndexOptions=Index vector (dialog)  Indices=[2]  OutputSizes=1
  Sum : Sum  Inputs=|++
  Position : Outport
  Orientation : Outport  Port=2
  wires:
  Sum/1 -> Matrix Concatenate/4
  Constant2/1 -> Matrix Concatenate/1
  Constant3/1 -> Matrix Concatenate1/2
  Gain/1 -> Matrix Concatenate1/3
  Constant4/1 -> Sum/2
  Constant1/1 -> Matrix Concatenate/2
  Selector1/1 -> Sum/1
  Constant/1 -> Matrix Concatenate/3
  Matrix Concatenate/1 -> Orientation/1
  Matrix Concatenate1/1 -> Position/1
  Selector4/1 -> Gain/1
  Selector3/1 -> Matrix Concatenate1/1
  Pose/1 -> Selector1/1, Selector4/1, Selector3/1

== system MOBATSim/Vehicle Model 5/Vehicle Model - Kinematic 3DOF Single Track ==
  WhlAngF : Inport
  xdotin : Inport  Port=2
  Delay : Delay  DelayLength=1  SampleTime=Sim_Ts
  Kinematic Bicycle Model : Subsystem
  Selector3 : Selector  InputPortWidth=3  IndexOptions=Index vector (dialog)  Indices=[1]  OutputSizes=1
  Selector4 : Selector  InputPortWidth=3  IndexOptions=Index vector (dialog)  Indices=[2]  OutputSizes=1
  Sqrt : Sqrt  SaturateOnIntegerOverflow=on
  Square : Math  Operator=square  SaturateOnIntegerOverflow=on
  Square1 : Math  Operator=square  SaturateOnIntegerOverflow=on
  Sum1 : Sum  Inputs=|++
  Zero-Order Hold1 : ZeroOrderHold  SampleTime=Sim_Ts
  Zero-Order Hold2 : ZeroOrderHold  SampleTime=Sim_Ts
  Pose : Outport
  xdot : Outport  Port=2
  wires:
  WhlAngF/1 -> Kinematic Bicycle Model/2(Steering Angle)
  xdotin/1 -> Kinematic Bicycle Model/1(v)
  Kinematic Bicycle Model/2(stateDot) -> Zero-Order Hold2/1
  Selector3/1 -> Square/1
  Sum1/1 -> Sqrt/1
  Square1/1 -> Sum1/2
  Selector4/1 -> Square1/1
  Sqrt/1 -> Delay/1
  Square/1 -> Sum1/1
  Delay/1 -> xdot/1
  Kinematic Bicycle Model/1(state) -> Zero-Order Hold1/1
  Zero-Order Hold1/1 -> Pose/1
  Zero-Order Hold2/1 -> Selector3/1, Selector4/1
